simulink model "ask_demod"  (R2018a)
settings: Solver=VariableStepAuto  StartTime=0.0  StopTime=10  RelTol=1e-3
libraries: commrandsrc3 x1
settings Model: Creator=hp  LastModifiedBy=hp

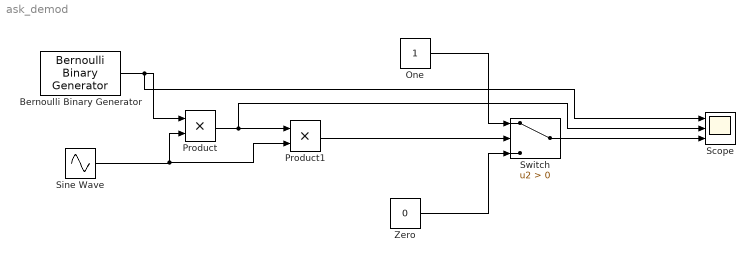
== system ask_demod ==
  Bernoulli Binary Generator : commrandsrc3/Bernoulli Binary Generator  ProbabilityOfZero=0.5  SeedSource=Auto  Seed=0  SampleTime=1  SamplesPerFrame=1  OutputDataType=double  SimulateUsing=Interpreted execution
  One : Constant
  Product : Product
  Product1 : Product
  Scope : Scope  NumInputPorts=3
  Sine Wave : Sin  SampleTime=0
  Switch : Switch  Criteria=u2 > Threshold
  Zero : Constant  Value=0
  wires:
  Bernoulli Binary Generator/1 -> Scope/1, Product/1
  Sine Wave/1 -> Product1/2, Product/2
  Product/1 -> Scope/2, Product1/1
  Zero/1 -> Switch/3
  One/1 -> Switch/1
  Switch/1 -> Scope/3
  Product1/1 -> Switch/2
